simulink model "Rectangular_polar"  (R2020a)
settings: Solver=VariableStepAuto  StartTime=0.0  StopTime=10.0  RelTol=1e-3
settings Model: Creator=royde  LastModifiedBy=royde

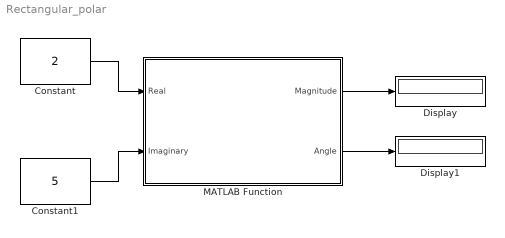
== system Rectangular_polar ==
  "Constant " : Constant  Value=2
  Constant1 : Constant  Value=5
  Display : Display
  Display1 : Display
  MATLAB Function : MATLAB Function  TreatAsAtomicUnit=on
  wires:
  "Constant "/1 -> MATLAB Function/1(Real)
  Constant1/1 -> MATLAB Function/2(Imaginary)
  MATLAB Function/2(Angle) -> Display1/1
  MATLAB Function/1(Magnitude) -> Display/1

== matlab function Rectangular_polar/MATLAB Function ==
  data: Real input; Magnitude output; Angle output; Imaginary input
function [Magnitude, Angle] = Rectangular_to_polar(Real, Imaginary)
Magnitude = sqrt(Real^2 + Imaginary^2);
Angle = atan(Imaginary/Real)*(180/pi);
